simulink library "Power_Shaft2_Ideal_A1_A2"  (R2026a)
settings: Solver=VariableStepAuto
undefined symbols (not defined in the file): ShaftA1, ShaftA2
libraries: fl_lib x3, Power_Components x2, nesl_utility x2, sm_lib x1
Description:
  | Component of Simscape Vehicle Templates Library
  | 
  | Copyright 2018-2026 The MathWorks, Inc.
settings Model: Creator=smiller  LastModifiedBy=smiller

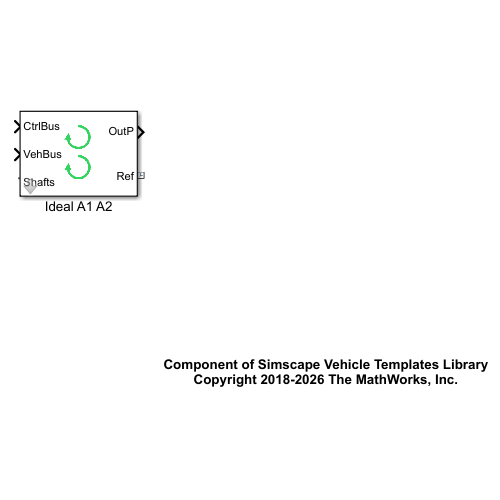
[thumbnail: Simulink's stored preview of the top-level diagram]
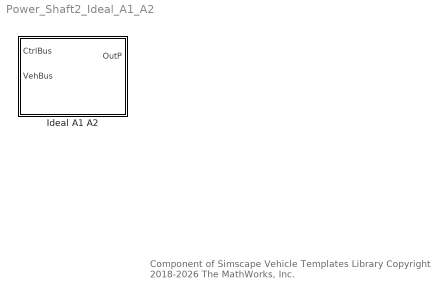
== system Power_Shaft2_Ideal_A1_A2 ==
  note: Component of Simscape Vehicle Templates Library
      | Copyright 2018-2026 The MathWorks, Inc.
  Ideal A1 A2 : Subsystem  VariantControl=IdealTwoMotor  mask(Two Ideal Motors, Axles 1 and 2){motor_ts_a1=100, motor_ts_a2=100}
      mask prompts: motor_ts_a1 "Axle 1 Motor Cutoff Frequency (Hz)"; motor_ts_a2 "Axle 2 Motor Cutoff Frequency (Hz)"
      mask help: Models two ideal motors connected to first and second axles in vehicle driveline.
      mask Display: image('sm_car_vehicle_power_ideal2motor_IMAGE.png');

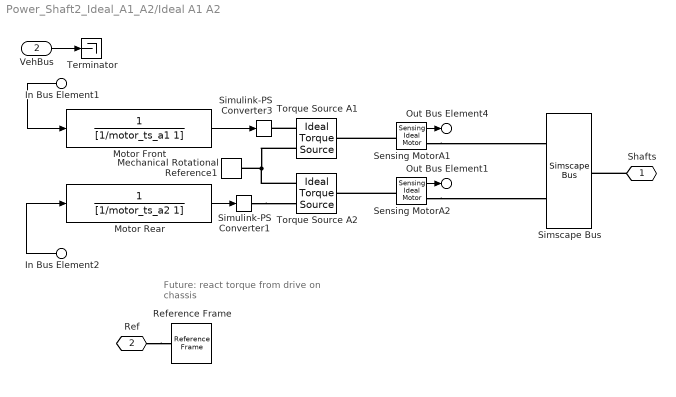
== system Power_Shaft2_Ideal_A1_A2/Ideal A1 A2 ==
  note: Future: react torque from
      | drive on chassis
  In Bus Element1 : Inport  PortName=CtrlBus  Element=MMotorA1Demand
  In Bus Element2 : Inport  PortName=CtrlBus  Element=MMotorA2Demand
  VehBus : Inport  Port=2
  Mechanical Rotational Reference1 : fl_lib/Mechanical/Rotational Elements/Mechanical Rotational Reference
  Motor Front : TransferFcn  Denominator=[1/motor_ts_a1 1]
  Motor Rear : TransferFcn  Denominator=[1/motor_ts_a2 1]
  Reference Frame : sm_lib/Frames and Transforms/Reference Frame
  Sensing MotorA1 : Power_Components/Sensing Ideal Motor  SystemSampleTime=-1  VariantActivationTime=update diagram  EmptyChoice=off  PassThrough=off  PassThroughVariantControl=(default)  EmptyChoiceVariantControl=(default)  AllowFlexibleInterface=on  Latency=0  AutoFrameSizeCalculation=off
  Sensing MotorA2 : Power_Components/Sensing Ideal Motor  SystemSampleTime=-1  VariantActivationTime=update diagram  EmptyChoice=off  PassThrough=off  PassThroughVariantControl=(default)  EmptyChoiceVariantControl=(default)  AllowFlexibleInterface=on  Latency=0  AutoFrameSizeCalculation=off
  Simscape Bus : SimscapeBus  HierarchyStrings=ShaftA1;ShaftA2
  Simulink-PS Converter1 : nesl_utility/Simulink-PS Converter  PhysicalDomain=network_engine_domain  SubClassName=ps_input  LeftPortType=input  RightPortType=output  PseudoPeriodic=off  Frequencies=[]  NoiseDistribution=none  NoiseParameters=[]  Unit=1  AffineConversion=off  FilteringAndDerivatives=provide  SimscapeFilterOrder=1  InputFilterTimeConstant=0.001  UdotUserProvided=0
  Simulink-PS Converter3 : nesl_utility/Simulink-PS Converter  PhysicalDomain=network_engine_domain  SubClassName=ps_input  LeftPortType=input  RightPortType=output  PseudoPeriodic=off  Frequencies=[]  NoiseDistribution=none  NoiseParameters=[]  Unit=1  AffineConversion=off  FilteringAndDerivatives=provide  SimscapeFilterOrder=1  InputFilterTimeConstant=0.001  UdotUserProvided=0
  Terminator : Terminator
  Torque Source A1 : fl_lib/Mechanical/Mechanical Sources/Ideal Torque Source
  Torque Source A2 : fl_lib/Mechanical/Mechanical Sources/Ideal Torque Source
  Shafts : PMIOPort  Side=Left
  Ref : PMIOPort  Port=2  Side=Right
  Out Bus Element4 : Outport  VectorParamsAs1DForOutWhenUnconnected=off  PortName=OutP  Element=MotorA1
  Out Bus Element1 : Outport  VectorParamsAs1DForOutWhenUnconnected=off  PortName=OutP  Element=MotorA2
  wires:
  Motor Rear/1 -> Simulink-PS Converter1/1
  Motor Front/1 -> Simulink-PS Converter3/1
  In Bus Element1/1 -> Motor Front/1
  In Bus Element2/1 -> Motor Rear/1
  VehBus/1 -> Terminator/1
  Sensing MotorA1/1 -> Out Bus Element4/1
  Sensing MotorA2/1 -> Out Bus Element1/1
  connections:
  Sensing MotorA2/RConn1 -- Simscape Bus/LConn2
  Sensing MotorA1/RConn1 -- Simscape Bus/LConn1
  Ref/RConn1 -- Reference Frame/RConn1
  Shafts/RConn1 -- Simscape Bus/RConn1
  Torque Source A2/RConn2 -- Mechanical Rotational Reference1/LConn1 -- Torque Source A1/RConn2
  Simulink-PS Converter1/RConn1 -- Torque Source A2/RConn1
  Torque Source A1/RConn1 -- Simulink-PS Converter3/RConn1
  Sensing MotorA1/LConn1 -- Torque Source A1/LConn1
  Sensing MotorA2/LConn1 -- Torque Source A2/LConn1
